simulink model "Main"  (R2017b)
settings: Solver=VariableStepAuto  StartTime=0.0  StopTime=100  FixedStep=0.00001  RelTol=1e-3
InitFcn:
  | Ku=1038641.6;
  | Tu=0.0054;
libraries: simulink x1
settings Model: Creator=Saadatyar  LastModifiedBy=rsaad

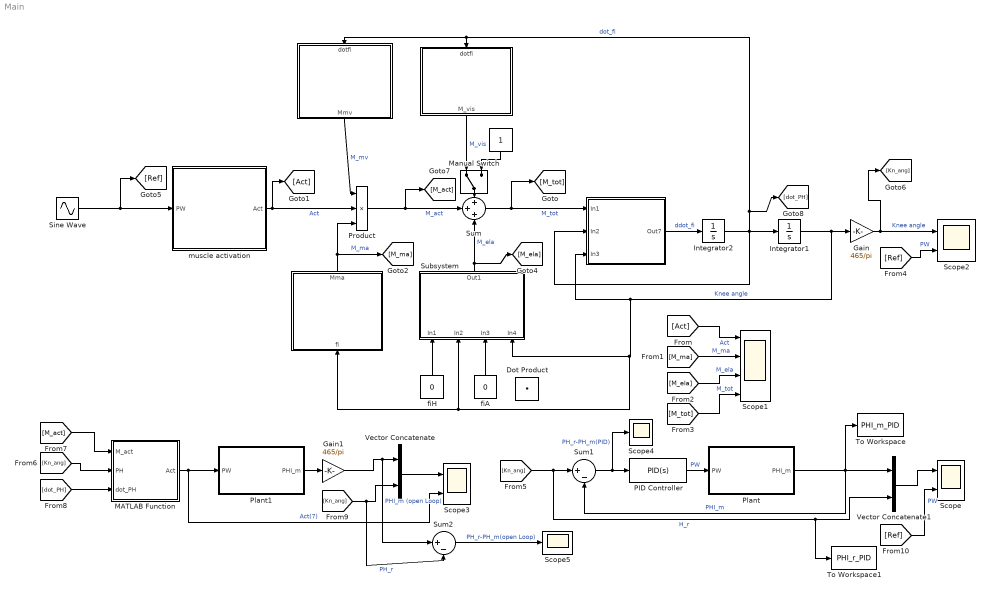
== system Main ==
  " " : MATLAB Function  TreatAsAtomicUnit=on
  " " : Constant
  " " : Subsystem
      mask Display: image(imread('1.JPG'));
  " " : MATLAB Function  TreatAsAtomicUnit=on
  " " : MATLAB Function  TreatAsAtomicUnit=on
  Dot Product : DotProduct  InputSameDT=on  OutDataTypeStr=Inherit: Inherit via internal rule
  Gain : Gain  Gain=465/pi
  Gain1 : Gain  Gain=465/pi
  Integrator1 : Integrator  InitialCondition=0.9
  Integrator2 : Integrator  InitialCondition=1.8
  MATLAB Function : MATLAB Function  TreatAsAtomicUnit=on
  Manual Switch : ManualSwitch
  PID Controller : simulink/Continuous/PID Controller  Controller=PID  TimeDomain=Continuous-time  SampleTime=-1  IntegratorMethod=Forward Euler  FilterMethod=Forward Euler  Form=Parallel  UseFilter=on  ControllerParametersSource=internal  P=0.6*Ku  I=1.2*Ku*Tu  D=0.6*Ku*Tu/8  N=1000  InitialConditionSource=internal  InitialConditionForIntegrator=0  InitialConditionForFilter=0  ExternalReset=none  LimitOutput=off  UpperSaturationLimit=inf  LowerSaturationLimit=-inf  LinearizeAsGain=on  AntiWindupMode=none  Kb=1  TrackingMode=off  Kt=1  PParamMin=[]  PParamMax=[]  IParamMin=[]  IParamMax=[]  DParamMin=[]  DParamMax=[]  NParamMin=[]  NParamMax=[]  KbParamMin=[]  KbParamMax=[]  KtParamMin=[]  KtParamMax=[]  POutMin=[]  POutMax=[]  IOutMin=[]  IOutMax=[]  DOutMin=[]  DOutMax=[]  NOutMin=[]  NOutMax=[]  KbOutMin=[]  KbOutMax=[]  KtOutMin=[]  KtOutMax=[]  IntegratorOutMin=[]  IntegratorOutMax=[]  FilterOutMin=[]  FilterOutMax=[]  SumOutMin=[]  SumOutMax=[]  SumI1OutMin=[]  SumI1OutMax=[]  SumI2OutMin=[]  SumI2OutMax=[]  SumI3OutMin=[]  SumI3OutMax=[]  SumDOutMin=[]  SumDOutMax=[]  SaturationOutMin=[]  SaturationOutMax=[]  IntegratorContinuousStateAttributes=''  IntegratorStateMustResolveToSignalObject=off  IntegratorRTWStateStorageClass=Auto  FilterContinuousStateAttributes=''  FilterStateMustResolveToSignalObject=off  FilterRTWStateStorageClass=Auto  DifferentiatorICPrevScaledInput=0  DifferentiatorOutMin=[]  DifferentiatorOutMax=[]  InitialConditionSetting=State (most efficient)  FilterDiffOutCoefMin=[]  FilterDiffOutCoefMax=[]  SumDenOutMin=[]  SumDenOutMax=[]  SumNumOutMin=[]  SumNumOutMax=[]  ReciprocalOutMin=[]  ReciprocalOutMax=[]  DivideOutMin=[]  DivideOutMax=[]  TunerSelectOption=Transfer Function Based (PID Tuner App)
  Plant : Subsystem
  Plant1 : Subsystem
  Product : Product  Inputs=3
  Scope : Scope  NumInputPorts=2
  Scope1 : Scope  NumInputPorts=4
  Scope2 : Scope  NumInputPorts=2
  Scope3 : Scope  NumInputPorts=2
  Scope4 : Scope
  Scope5 : Scope
  Sine Wave : Sin  Amplitude=100  Bias=150  Frequency=1.5707  Samples=31.38  SampleTime=0.04  VectorParams1D=off
  Subsystem : Subsystem
      mask Display: image(imread('5.JPG'));
  Sum : Sum  Inputs=+++
  Sum1 : Sum  Inputs=|+-
  Sum2 : Sum  Inputs=|+-
  To Workspace : ToWorkspace  VariableName=PHI_m_PID  SampleTime=-1
      settings: Save2DSignal=2-D array (concatenate along first dimension)
  To Workspace1 : ToWorkspace  VariableName=PHI_r_PID  SampleTime=-1
      settings: Save2DSignal=2-D array (concatenate along first dimension)
  Vector Concatenate : Concatenate
  Vector Concatenate1 : Concatenate
  fiA : Constant  Value=0
  fiH : Constant  Value=0
  "muscle activation " : MATLAB Function  TreatAsAtomicUnit=on
  wires:
  " "/1(Mmv) -> Product/1  "M_mv"
  "muscle activation "/1(Act) -> Product/2, [Act]  "Act"
  " "/1(Mma) -> [M_ma], Product/3  "M_ma"
  Product/1 -> [M_act], Sum/2  "M_act"
  " "/1(M_vis) -> Manual Switch/1  "M_vis"
  fiH/1 -> Subsystem/1(In1)
  fiA/1 -> Subsystem/3(In3)
  Subsystem/1(Out1) -> [M_ela], Sum/3  "M_ela"
  Manual Switch/1 -> Sum/1
  " "/1 -> Manual Switch/2
  Sum/1 -> [M_tot], " "/1("In1 ")  "M_tot"
  " "/1(Out7) -> Integrator2/1  "ddot_fi"
  Integrator2/1 -> [dot_PH], " "/1(dotfi), " "/1(dotfi), " "/2(In2), Integrator1/1  "dot_fi"
  Integrator1/1 -> Gain/1, " "/1(fi), Subsystem/2(In2), Subsystem/4(In4), " "/3(In3)  "Knee angle"
  [Act] -> Scope1/1  "Act"
  [M_ma] -> Scope1/2  "M_ma"
  [M_ela] -> Scope1/3  "M_ela"
  [M_tot] -> Scope1/4  "M_tot"
  Sine Wave/1 -> [Ref], "muscle activation "/1(PW)
  [Ref] -> Scope2/2  "PW"
  Gain/1 -> [Kn_ang], Scope2/1  "Knee angle"
  [M_act] -> MATLAB Function/1(M_act)
  [dot_PH] -> MATLAB Function/3(dot_PH)
  [Kn_ang] -> MATLAB Function/2(PH)
  MATLAB Function/1(Act) -> Scope3/2, Plant1/1(PW)  "Act(7)"
  Plant/1(PHI_m) -> To Workspace/1, Sum1/2, Vector Concatenate1/1  "PHI_m"
  PID Controller/1 -> Plant/1(PW)  "PW"
  Sum1/1 -> Scope4/1, PID Controller/1  "PH_r-PH_m(PID)"
  [Kn_ang] -> To Workspace1/1, Vector Concatenate1/2, Sum1/1  "H_r"
  Plant1/1(PHI_m) -> Gain1/1
  Gain1/1 -> Sum2/1, Vector Concatenate/1  "PHI_m (open Loop)"
  [Kn_ang] -> Sum2/2, Vector Concatenate/2  "PH_r"
  Vector Concatenate/1 -> Scope3/1
  Vector Concatenate1/1 -> Scope/1
  [Ref] -> Scope/2  "PW"
  Sum2/1 -> Scope5/1  "PH_r-PH_m(open Loop)"

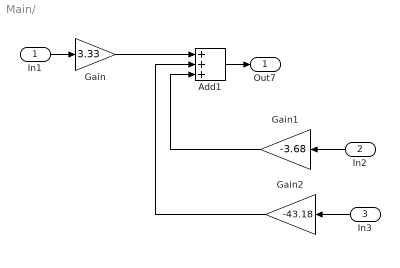
== system Main/  ==
  "In1 " : Inport
  In2 : Inport  Port=2
  In3 : Inport  Port=3
  Add1 : Sum  Inputs=+++
  Gain : Gain  Gain=3.33
  Gain1 : Gain  Gain=-3.68
  Gain2 : Gain  Gain=-43.18
  Out7 : Outport
  wires:
  Gain1/1 -> Add1/3
  Gain2/1 -> Add1/2
  Gain/1 -> Add1/1
  In2/1 -> Gain1/1
  In3/1 -> Gain2/1
  "In1 "/1 -> Gain/1
  Add1/1 -> Out7/1

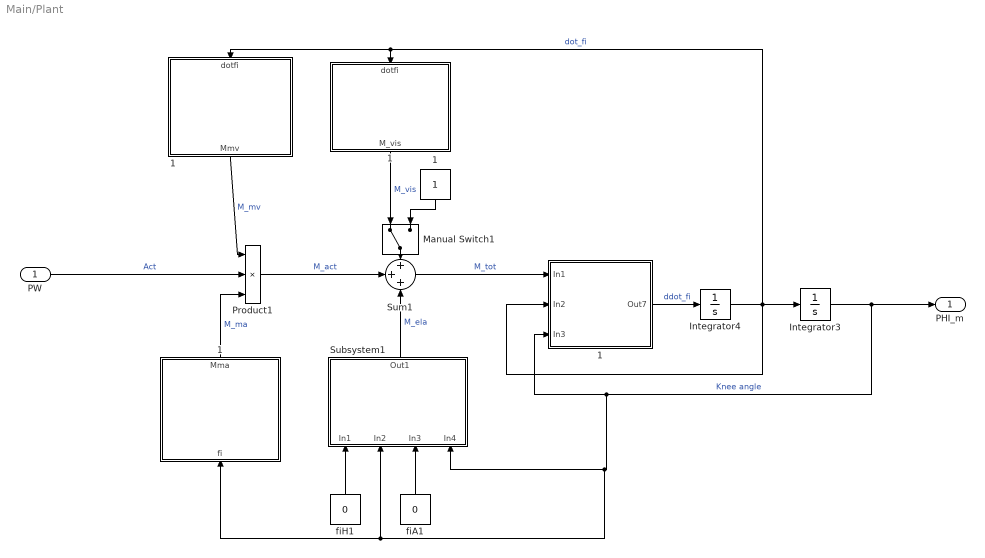
== system Main/Plant ==
  PW : Inport
  " 1" : MATLAB Function  TreatAsAtomicUnit=on
  " 1" : Subsystem
      mask Display: image(imread('1.JPG'));
  " 1" : Constant
  " 1" : MATLAB Function  TreatAsAtomicUnit=on
  " 1" : MATLAB Function  TreatAsAtomicUnit=on
  Integrator3 : Integrator  InitialCondition=0.9
  Integrator4 : Integrator  InitialCondition=1.8
  Manual Switch1 : ManualSwitch
  Product1 : Product  Inputs=3
  Subsystem1 : Subsystem
      mask Display: image(imread('5.JPG'));
  Sum1 : Sum  Inputs=+++
  fiA1 : Constant  Value=0
  fiH1 : Constant  Value=0
  PHI_m : Outport
  wires:
  fiA1/1 -> Subsystem1/3(In3)
  Integrator3/1 -> PHI_m/1, " 1"/1(fi), Subsystem1/2(In2), Subsystem1/4(In4), " 1"/3(In3)  "Knee angle"
  " 1"/1(M_vis) -> Manual Switch1/1  "M_vis"
  Subsystem1/1(Out1) -> Sum1/3  "M_ela"
  " 1"/1(Mma) -> Product1/3  "M_ma"
  PW/1 -> Product1/2  "Act"
  " 1"/1(Mmv) -> Product1/1  "M_mv"
  Integrator4/1 -> " 1"/1(dotfi), " 1"/1(dotfi), " 1"/2(In2), Integrator3/1  "dot_fi"
  " 1"/1 -> Manual Switch1/2
  Product1/1 -> Sum1/2  "M_act"
  Manual Switch1/1 -> Sum1/1
  Sum1/1 -> " 1"/1("In1 ")  "M_tot"
  " 1"/1(Out7) -> Integrator4/1  "ddot_fi"
  fiH1/1 -> Subsystem1/1(In1)

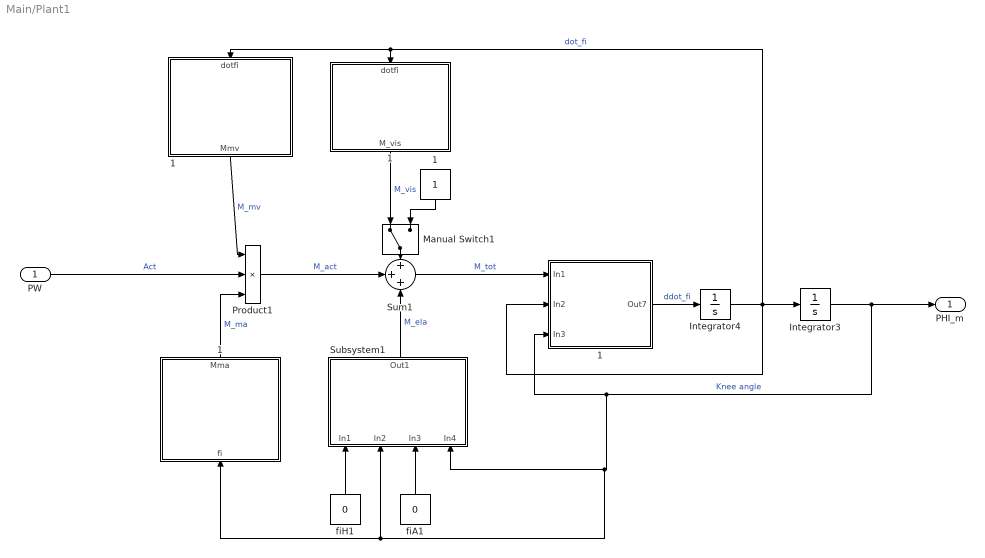
== system Main/Plant1 ==
  PW : Inport
  " 1" : MATLAB Function  TreatAsAtomicUnit=on
  " 1" : Subsystem
      mask Display: image(imread('1.JPG'));
  " 1" : Constant
  " 1" : MATLAB Function  TreatAsAtomicUnit=on
  " 1" : MATLAB Function  TreatAsAtomicUnit=on
  Integrator3 : Integrator  InitialCondition=0.9
  Integrator4 : Integrator  InitialCondition=1.8
  Manual Switch1 : ManualSwitch
  Product1 : Product  Inputs=3
  Subsystem1 : Subsystem
      mask Display: image(imread('5.JPG'));
  Sum1 : Sum  Inputs=+++
  fiA1 : Constant  Value=0
  fiH1 : Constant  Value=0
  PHI_m : Outport
  wires:
  fiA1/1 -> Subsystem1/3(In3)
  Integrator3/1 -> PHI_m/1, " 1"/1(fi), Subsystem1/2(In2), Subsystem1/4(In4), " 1"/3(In3)  "Knee angle"
  " 1"/1(M_vis) -> Manual Switch1/1  "M_vis"
  Subsystem1/1(Out1) -> Sum1/3  "M_ela"
  " 1"/1(Mma) -> Product1/3  "M_ma"
  PW/1 -> Product1/2  "Act"
  " 1"/1(Mmv) -> Product1/1  "M_mv"
  Integrator4/1 -> " 1"/1(dotfi), " 1"/1(dotfi), " 1"/2(In2), Integrator3/1  "dot_fi"
  " 1"/1 -> Manual Switch1/2
  Product1/1 -> Sum1/2  "M_act"
  Manual Switch1/1 -> Sum1/1
  Sum1/1 -> " 1"/1("In1 ")  "M_tot"
  " 1"/1(Out7) -> Integrator4/1  "ddot_fi"
  fiH1/1 -> Subsystem1/1(In1)

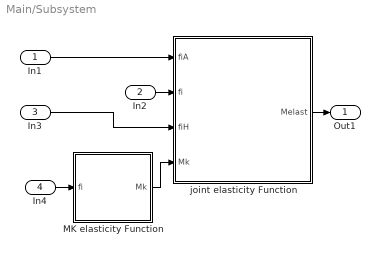
== system Main/Subsystem ==
  In1 : Inport
  In2 : Inport  Port=2
  In3 : Inport  Port=3
  In4 : Inport  Port=4
  MK elasticity Function : MATLAB Function  TreatAsAtomicUnit=on
  joint elasticity Function : MATLAB Function  TreatAsAtomicUnit=on
  Out1 : Outport
  wires:
  MK elasticity Function/1(Mk) -> joint elasticity Function/4(Mk)
  In1/1 -> joint elasticity Function/1(fiA)
  In3/1 -> joint elasticity Function/3(fiH)
  In4/1 -> MK elasticity Function/1(fi)
  joint elasticity Function/1(Melast) -> Out1/1
  In2/1 -> joint elasticity Function/2(fi)

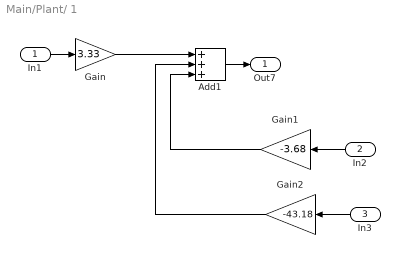
== system Main/Plant/ 1 ==
  "In1 " : Inport
  In2 : Inport  Port=2
  In3 : Inport  Port=3
  Add1 : Sum  Inputs=+++
  Gain : Gain  Gain=3.33
  Gain1 : Gain  Gain=-3.68
  Gain2 : Gain  Gain=-43.18
  Out7 : Outport
  wires:
  Gain1/1 -> Add1/3
  Gain2/1 -> Add1/2
  Gain/1 -> Add1/1
  In2/1 -> Gain1/1
  In3/1 -> Gain2/1
  "In1 "/1 -> Gain/1
  Add1/1 -> Out7/1

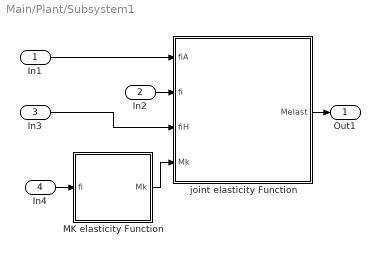
== system Main/Plant/Subsystem1 ==
  In1 : Inport
  In2 : Inport  Port=2
  In3 : Inport  Port=3
  In4 : Inport  Port=4
  MK elasticity Function : MATLAB Function  TreatAsAtomicUnit=on
  joint elasticity Function : MATLAB Function  TreatAsAtomicUnit=on
  Out1 : Outport
  wires:
  MK elasticity Function/1(Mk) -> joint elasticity Function/4(Mk)
  In1/1 -> joint elasticity Function/1(fiA)
  In3/1 -> joint elasticity Function/3(fiH)
  In4/1 -> MK elasticity Function/1(fi)
  joint elasticity Function/1(Melast) -> Out1/1
  In2/1 -> joint elasticity Function/2(fi)

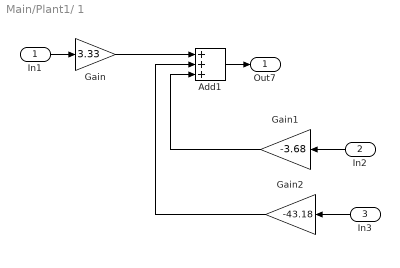
== system Main/Plant1/ 1 ==
  "In1 " : Inport
  In2 : Inport  Port=2
  In3 : Inport  Port=3
  Add1 : Sum  Inputs=+++
  Gain : Gain  Gain=3.33
  Gain1 : Gain  Gain=-3.68
  Gain2 : Gain  Gain=-43.18
  Out7 : Outport
  wires:
  Gain1/1 -> Add1/3
  Gain2/1 -> Add1/2
  Gain/1 -> Add1/1
  In2/1 -> Gain1/1
  In3/1 -> Gain2/1
  "In1 "/1 -> Gain/1
  Add1/1 -> Out7/1

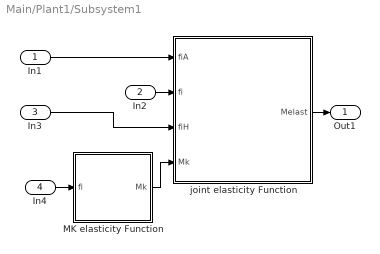
== system Main/Plant1/Subsystem1 ==
  In1 : Inport
  In2 : Inport  Port=2
  In3 : Inport  Port=3
  In4 : Inport  Port=4
  MK elasticity Function : MATLAB Function  TreatAsAtomicUnit=on
  joint elasticity Function : MATLAB Function  TreatAsAtomicUnit=on
  Out1 : Outport
  wires:
  MK elasticity Function/1(Mk) -> joint elasticity Function/4(Mk)
  In1/1 -> joint elasticity Function/1(fiA)
  In3/1 -> joint elasticity Function/3(fiH)
  In4/1 -> MK elasticity Function/1(fi)
  joint elasticity Function/1(Melast) -> Out1/1
  In2/1 -> joint elasticity Function/2(fi)

== matlab function Main/  ==
  data: fi input; Mma output
function Mma = fcn(fi)
k1=60;
k2=65;
 Mma= exp(-((fi-k1)/k2)^2);

== matlab function Main/muscle activation  ==
  data: PW input; Act output
function Act=fcn(PW)
Sf=15;
Thres=100;
Sat=500;
if  PW<=Thres
    Act=0;
elseif (Thres<PW) && (PW<Sat)
    Act=(Sf/(Sat-Thres))*(PW-Thres);
else
    Act=Sf;
end
end

== matlab function Main/  ==
  data: Mmv output; dotfi input
function Mmv= fcn(dotfi)
k3=0.04;
Mmv=1-(k3*dotfi);

== matlab function Main/Subsystem/MK elasticity Function ==
  data: fi input; Mk output
function Mk = fcn(fi)
Mk=exp(2.220-(0.150*fi));

== matlab function Main/Subsystem/joint elasticity Function ==
  data: fiA input; Melast output; fi input; fiH input; Mk input
function Melast = fcn(fiA,fi,fiH,Mk)
Melast = exp(1.800-(0.0460*fiA)+(0.0217*fiH)-(0.0352*fi))- exp(-3.971-(0.0004*fiA)-(0.0495*fi)-(0.0128*fiH))-4.820+Mk;

== matlab function Main/Plant/ 1 ==
  data: fi input; Mma output
function Mma = fcn(fi)
k1=60;
k2=65;
 Mma= exp(-((fi-k1)/k2)^2);

== matlab function Main/Plant/ 1 ==
  data: dotfi input; M_vis output
function M_vis = fcn(dotfi)
M_vis=-0.86*dotfi;

== matlab function Main/  ==
  data: dotfi input; M_vis output
function M_vis = fcn(dotfi)
M_vis=-0.86*dotfi;

== matlab function Main/Plant/ 1 ==
  data: Mmv output; dotfi input
function Mmv= fcn(dotfi)
k3=0.04;
Mmv=1-(k3*dotfi);

== matlab function Main/Plant/Subsystem1/MK elasticity Function ==
  data: fi input; Mk output
function Mk = fcn(fi)
Mk=exp(2.220-(0.150*fi));

== matlab function Main/Plant/Subsystem1/joint elasticity Function ==
  data: fiA input; Melast output; fi input; fiH input; Mk input
function Melast = fcn(fiA,fi,fiH,Mk)
Melast = exp(1.800-(0.0460*fiA)+(0.0217*fiH)-(0.0352*fi))- exp(-3.971-(0.0004*fiA)-(0.0495*fi)-(0.0128*fiH))-4.820+Mk;

== matlab function Main/Plant1/ 1 ==
  data: fi input; Mma output
function Mma = fcn(fi)
k1=60;
k2=65;
 Mma= exp(-((fi-k1)/k2)^2);

== matlab function Main/MATLAB Function ==
  data: M_act input; Act output; PH input; dot_PH input
function Act = fcn(M_act,PH,dot_PH)
k1=60;
k2=65;
k3=0.04;
Act=(M_act*exp(((PH-k1)/k2)^2))/(1-k3*dot_PH);

== matlab function Main/Plant1/ 1 ==
  data: dotfi input; M_vis output
function M_vis = fcn(dotfi)
M_vis=-0.86*dotfi;

== matlab function Main/Plant1/ 1 ==
  data: Mmv output; dotfi input
function Mmv= fcn(dotfi)
k3=0.04;
Mmv=1-(k3*dotfi);

== matlab function Main/Plant1/Subsystem1/MK elasticity Function ==
  data: fi input; Mk output
function Mk = fcn(fi)
Mk=exp(2.220-(0.150*fi));

== matlab function Main/Plant1/Subsystem1/joint elasticity Function ==
  data: fiA input; Melast output; fi input; fiH input; Mk input
function Melast = fcn(fiA,fi,fiH,Mk)
Melast = exp(1.800-(0.0460*fiA)+(0.0217*fiH)-(0.0352*fi))- exp(-3.971-(0.0004*fiA)-(0.0495*fi)-(0.0128*fiH))-4.820+Mk;
